simulink model "gnc"  (R2023a)
settings: Solver=ode4  StartTime=0.0  StopTime=10.0  FixedStep=dt  RelTol=1e-3
undefined symbols (not defined in the file): dt, plant, u_mat_full, u_time
libraries: aerolibutil x2
settings Model: Creator=ndelurgio  LastModifiedBy=ndelurgio

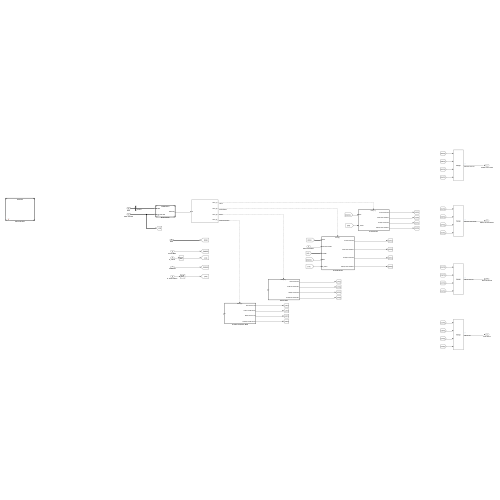
[thumbnail: Simulink's stored preview of the top-level diagram]
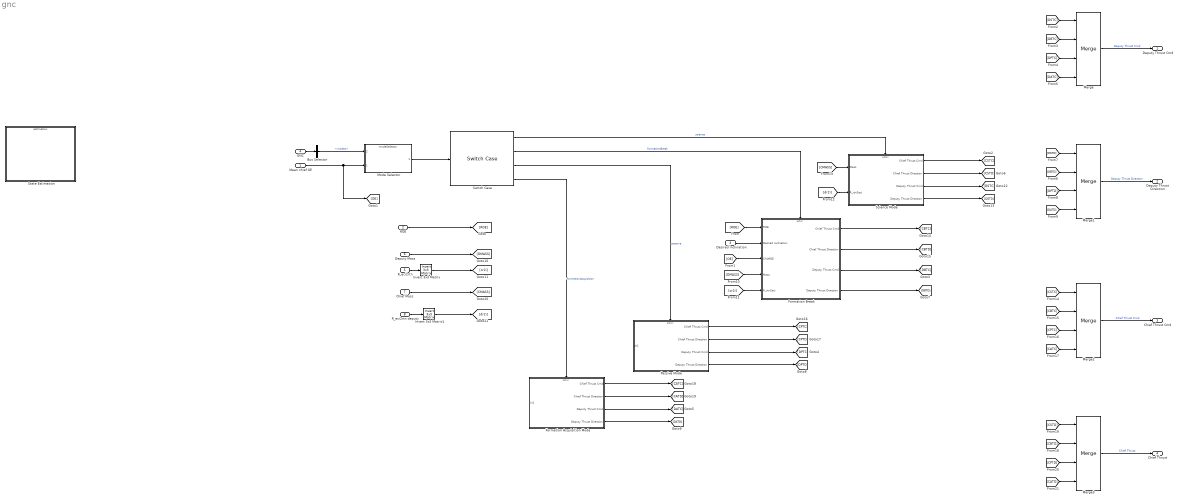
== system gnc ==
  Mean chief OE : Inport  OutDataTypeStr=Bus: meanOrbitElements
  ROE : Inport  Port=2  OutDataTypeStr=Bus: eccentricSingularROE
  Desired inclination : Inport  Port=3  PortDimensions=2
  GNC : Inport  Port=4  OutDataTypeStr=Bus: gncBus
  R_eci2rtn : Inport  Port=5  PortDimensions=[3,3]
  Deputy Mass : Inport  Port=6
  Chief Mass : Inport  Port=7
  R_eci2rtn deputy : Inport  Port=8
  Bus Selector : BusSelector  OutputSignals=modes
  Formation Acquisition Mode : Subsystem  TreatAsAtomicUnit=on
  Formation Break : Subsystem  TreatAsAtomicUnit=on
  Invert 3x3 Matrix : aerolibutil/Invert  3x3 Matrix
  Invert 3x3 Matrix1 : aerolibutil/Invert  3x3 Matrix
  Merge : Merge  Inputs=4  InitialOutput=0
  Merge1 : Merge  Inputs=4  InitialOutput=[1,1,1]
  Merge2 : Merge  Inputs=4  InitialOutput=0
  Merge3 : Merge  Inputs=4  InitialOutput=[1,1,1]
  Mode Selector : ModelReference  ModelNameDialog=modeSelector.slx  SimulationMode=Normal  ModelReferenceVersion=1.12
      settings: PortSchema="{\"entries\":[{\"content\":{\"sides\":[{\"content\":{\"connectorIds\":[\"In2\",\"In1\"]},\"type\":\"ConnectorPlacement.EquallySpacedRectSide\",\"uuid\":\"8a45dd05-9625-4267-a143-38565687985f\"},{\"content\":{\"connectorIds\":[\"Out1\"],\"side\":\"RIGHT\"},\"type\":\"ConnectorPlacement.EquallySpacedRectSide\",\"uuid\":\"c16609dd-c717-4d96-a97d-40d34aa61c5b\"},{\"content\":{\"side\":\"TOP\"},\"type\":\"ConnectorPlacement.EquallySpacedRectSide\",\"uuid\":\"265a618d-b5cc-4228-aeff-cbf882e13e2d\"}]},\"type\":\"ConnectorPlacement.EquallySpacedConnector\",\"uuid\":\"354b4fb0-049b-4d87-9ce4-a2a1b71aacc7\"}],\"packageUris\":[\"http://schema.mathworks.com/mf0/Connector/R2020b\"],\"version\":\"1.0\"}"
  Passive Mode : Subsystem  TreatAsAtomicUnit=on
  Science Mode : Subsystem  TreatAsAtomicUnit=on
  State Estimation : ModelReference  ModelNameDialog=estimation.slx  SimulationMode=Normal  ModelReferenceVersion=1.1
  Switch Case : SwitchCase  CaseConditions={1,2,3,4}  ShowDefaultCase=off
  Deputy Thrust Cmd : Outport
  Deputy Thrust Direction : Outport  Port=2
  Chief Thrust Cmd : Outport  Port=3
  Chief Thrust : Outport  Port=4
  wires:
  Mean chief OE/1 -> [OE], Mode Selector/1
  ROE/1 -> [ROE]
  Desired inclination/1 -> Formation Break/2(Desired inclination)
  Merge/1 -> Deputy Thrust Cmd/1  "Deputy Thrust Cmd"
  Merge1/1 -> Deputy Thrust Direction/1  "Deputy Thrust Direction"
  Switch Case/1 -> Science Mode/Action  "science"
  Switch Case/2 -> Formation Break/Action  "formationBreak"
  Switch Case/3 -> Passive Mode/Action  "passive"
  Switch Case/4 -> Formation Acquisition Mode/Action  "formationAcquisition"
  Mode Selector/1 -> Switch Case/1
  GNC/1 -> Bus Selector/1
  Bus Selector/1 -> Mode Selector/2  "<modes>"
  [ROE] -> Formation Break/1(ROE)
  [OE] -> Formation Break/3(ChiefOE)
  Invert 3x3 Matrix/1 -> [cr2i]
  Deputy Mass/1 -> [DMASS]
  R_eci2rtn/1 -> Invert 3x3 Matrix/1
  Science Mode/1(Chief Thrust Cmd) -> [CSTC]
  Formation Break/3(Deputy Thrust Cmd) -> [DBTC]
  Passive Mode/3(Deputy Thrust Cmd) -> [DPTC]
  Formation Acquisition Mode/3(Deputy Thrust Cmd) -> [DATC]
  [DSTC] -> Merge/1
  [DBTC] -> Merge/2
  [DPTC] -> Merge/3
  [DATC] -> Merge/4
  Science Mode/2(Chief Thrust Direction) -> [CSTD]
  Formation Break/4(Deputy Thrust Direction) -> [DBTD]
  Passive Mode/4(Deputy Thrust Direction) -> [DPTD]
  Formation Acquisition Mode/4(Deputy Thrust Direction) -> [DATD]
  [DSTD] -> Merge1/1
  [DBTD] -> Merge1/2
  [DPTD] -> Merge1/3
  [DATD] -> Merge1/4
  [DMASS] -> Formation Break/4(Mass)
  [cr2i] -> Formation Break/5(R_rtn2eci)
  [dr2i] -> Science Mode/2(R_rtn2eci)
  [CMASS] -> Science Mode/1(Mass)
  Science Mode/3(Deputy Thrust Cmd) -> [DSTC]
  Science Mode/4(Deputy Thrust Direction) -> [DSTD]
  Formation Break/2(Chief Thrust Direction) -> [CBTD]
  Formation Break/1(Chief Thrust Cmd) -> [CBTC]
  Passive Mode/1(Chief Thrust Cmd) -> [CPTC]
  Passive Mode/2(Chief Thrust Direction) -> [CPTD]
  Formation Acquisition Mode/1(Chief Thrust Cmd) -> [CATC]
  Formation Acquisition Mode/2(Chief Thrust Direction) -> [CATD]
  [CSTC] -> Merge2/1
  [CPTC] -> Merge2/3
  [CATC] -> Merge2/4
  [CBTC] -> Merge2/2
  [CSTD] -> Merge3/1
  [CBTD] -> Merge3/2
  [CATD] -> Merge3/4
  [CPTD] -> Merge3/3
  Merge3/1 -> Chief Thrust/1  "Chief Thrust"
  Merge2/1 -> Chief Thrust Cmd/1  "Chief Thrust Cmd"
  Chief Mass/1 -> [CMASS]
  R_eci2rtn deputy/1 -> Invert 3x3 Matrix1/1
  Invert 3x3 Matrix1/1 -> [dr2i]

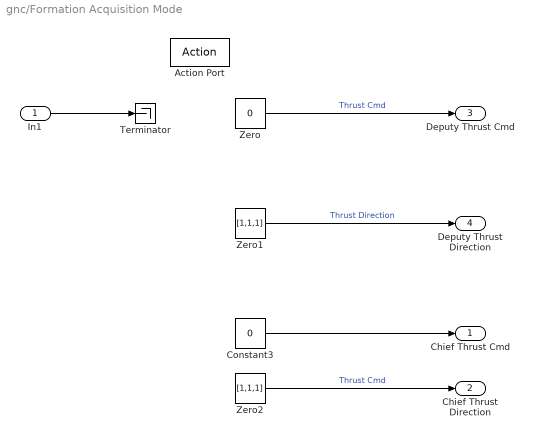
== system gnc/Formation Acquisition Mode ==
  In1 : Inport
  Action Port : ActionPort  ActionPortLabel=case [ 4 ]:
  Constant3 : Constant  Value=0
  Terminator : Terminator
  Zero : Constant  Value=0  OutDataTypeStr=Inherit: Inherit via back propagation
  Zero1 : Constant  Value=[1,1,1]  OutDataTypeStr=Inherit: Inherit via back propagation
  Zero2 : Constant  Value=[1,1,1]  OutDataTypeStr=Inherit: Inherit via back propagation
  Chief Thrust Cmd : Outport
  Chief Thrust Direction : Outport  Port=2
  Deputy Thrust Cmd : Outport  Port=3
  Deputy Thrust Direction : Outport  Port=4
  wires:
  In1/1 -> Terminator/1
  Zero/1 -> Deputy Thrust Cmd/1  "Thrust Cmd"
  Zero1/1 -> Deputy Thrust Direction/1  "Thrust Direction"
  Zero2/1 -> Chief Thrust Direction/1  "Thrust Cmd"
  Constant3/1 -> Chief Thrust Cmd/1

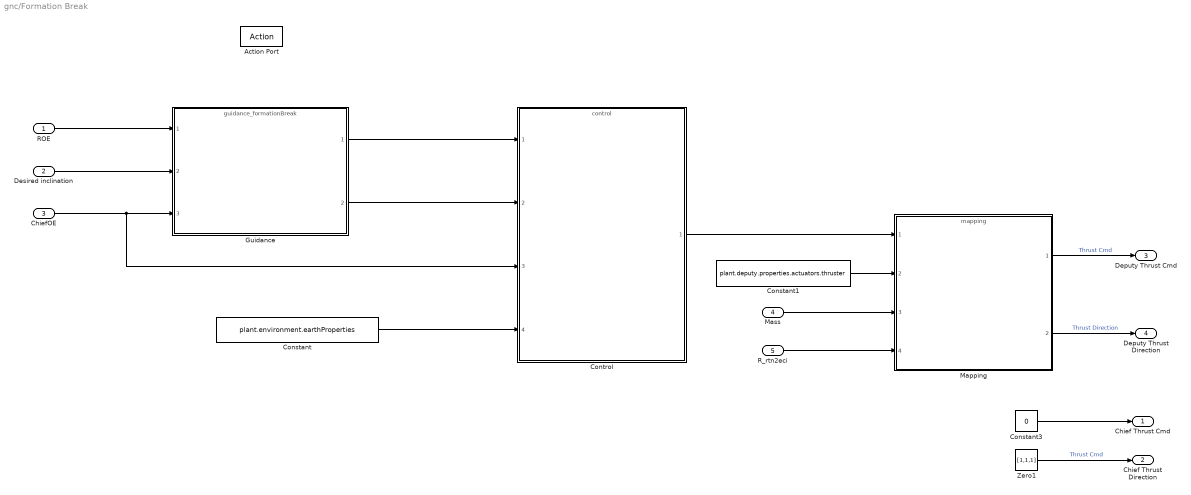
== system gnc/Formation Break ==
  ROE : Inport
  Desired inclination : Inport  Port=2
  ChiefOE : Inport  Port=3
  Mass : Inport  Port=4
  R_rtn2eci : Inport  Port=5
  Action Port : ActionPort  ActionPortLabel=case [ 2 ]:
  Constant : Constant  Value=plant.environment.earthProperties  OutDataTypeStr=Bus: earthProperties
  Constant1 : Constant  Value=plant.deputy.properties.actuators.thruster  OutDataTypeStr=Bus: thruster
  Constant3 : Constant  Value=0
  Control : ModelReference  ModelNameDialog=control.slx  SimulationMode=Normal  ModelReferenceVersion=1.13
  Guidance : ModelReference  ModelNameDialog=guidance_formationBreak  SimulationMode=Normal  ModelReferenceVersion=1.49
  Mapping : ModelReference  ModelNameDialog=mapping.slx  SimulationMode=Normal  ModelReferenceVersion=1.29
  Zero1 : Constant  Value=[1,1,1]  OutDataTypeStr=Inherit: Inherit via back propagation
  Chief Thrust Cmd : Outport
  Chief Thrust Direction : Outport  Port=2
  Deputy Thrust Cmd : Outport  Port=3
  Deputy Thrust Direction : Outport  Port=4
  wires:
  ROE/1 -> Guidance/1
  Guidance/1 -> Control/1
  Guidance/2 -> Control/2
  Desired inclination/1 -> Guidance/2
  ChiefOE/1 -> Control/3, Guidance/3
  Constant/1 -> Control/4
  Control/1 -> Mapping/1
  Constant1/1 -> Mapping/2
  Mass/1 -> Mapping/3
  R_rtn2eci/1 -> Mapping/4
  Mapping/1 -> Deputy Thrust Cmd/1  "Thrust Cmd"
  Mapping/2 -> Deputy Thrust Direction/1  "Thrust Direction"
  Constant3/1 -> Chief Thrust Cmd/1
  Zero1/1 -> Chief Thrust Direction/1  "Thrust Cmd"

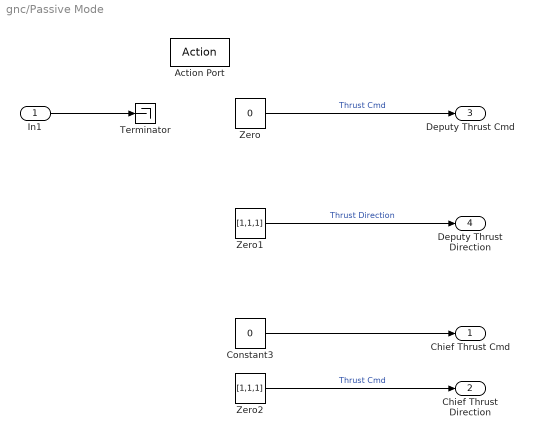
== system gnc/Passive Mode ==
  In1 : Inport
  Action Port : ActionPort  ActionPortLabel=case [ 3 ]:
  Constant3 : Constant  Value=0
  Terminator : Terminator
  Zero : Constant  Value=0  OutDataTypeStr=Inherit: Inherit via back propagation
  Zero1 : Constant  Value=[1,1,1]  OutDataTypeStr=Inherit: Inherit via back propagation
  Zero2 : Constant  Value=[1,1,1]  OutDataTypeStr=Inherit: Inherit via back propagation
  Chief Thrust Cmd : Outport
  Chief Thrust Direction : Outport  Port=2
  Deputy Thrust Cmd : Outport  Port=3
  Deputy Thrust Direction : Outport  Port=4
  wires:
  In1/1 -> Terminator/1
  Zero/1 -> Deputy Thrust Cmd/1  "Thrust Cmd"
  Zero1/1 -> Deputy Thrust Direction/1  "Thrust Direction"
  Zero2/1 -> Chief Thrust Direction/1  "Thrust Cmd"
  Constant3/1 -> Chief Thrust Cmd/1

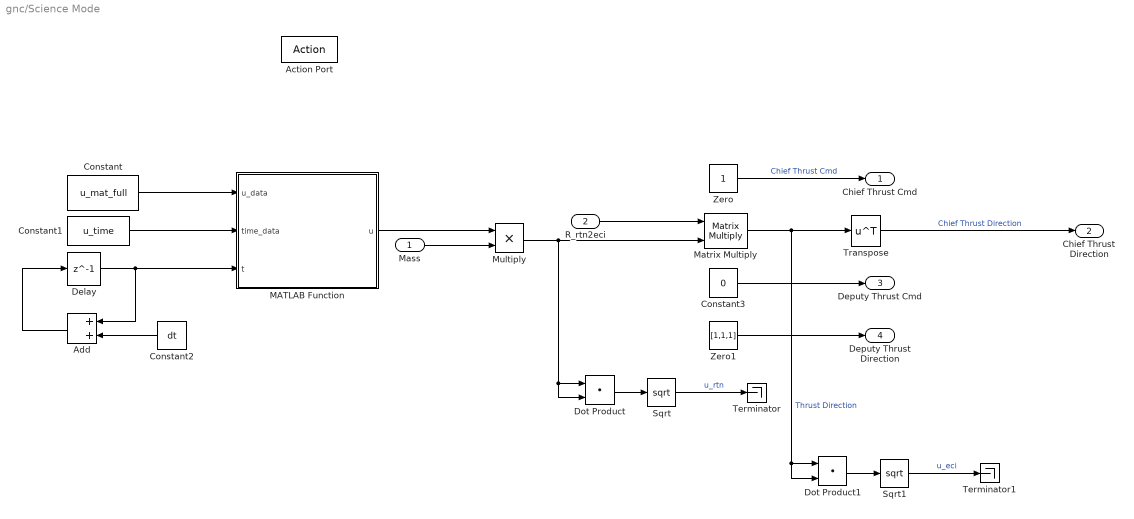
== system gnc/Science Mode ==
  Mass : Inport
  R_rtn2eci : Inport  Port=2
  Action Port : ActionPort  ActionPortLabel=case [ 1 ]:
  Add : Sum
  Constant : Constant  Value=u_mat_full
  Constant1 : Constant  Value=u_time
  Constant2 : Constant  Value=dt
  Constant3 : Constant  Value=0
  Delay : Delay  DelayLength=1
  Dot Product : DotProduct  OutDataTypeStr=Inherit: Inherit via internal rule
  Dot Product1 : DotProduct  OutDataTypeStr=Inherit: Inherit via internal rule
  MATLAB Function : MATLAB Function  TreatAsAtomicUnit=on
  Matrix Multiply : Product  Multiplication=Matrix(*)
  Multiply : Product  Inputs=**
  Sqrt : Sqrt
  Sqrt1 : Sqrt
  Terminator : Terminator
  Terminator1 : Terminator
  Transpose : Math  Operator=transpose
  Zero : Constant  OutDataTypeStr=Inherit: Inherit via back propagation
  Zero1 : Constant  Value=[1,1,1]  OutDataTypeStr=Inherit: Inherit via back propagation
  Chief Thrust Cmd : Outport
  Chief Thrust Direction : Outport  Port=2
  Deputy Thrust Cmd : Outport  Port=3
  Deputy Thrust Direction : Outport  Port=4
  wires:
  Zero/1 -> Chief Thrust Cmd/1  "Chief Thrust Cmd"
  Matrix Multiply/1 -> Dot Product1/2, Dot Product1/1, Transpose/1  "Thrust Direction"
  Constant/1 -> MATLAB Function/1(u_data)
  Constant1/1 -> MATLAB Function/2(time_data)
  Delay/1 -> Add/1, MATLAB Function/3(t)
  Constant2/1 -> Add/2
  Add/1 -> Delay/1
  MATLAB Function/1(u) -> Multiply/1
  Mass/1 -> Multiply/2
  R_rtn2eci/1 -> Matrix Multiply/1
  Multiply/1 -> Dot Product/2, Dot Product/1, Matrix Multiply/2
  Constant3/1 -> Deputy Thrust Cmd/1
  Zero1/1 -> Deputy Thrust Direction/1
  Transpose/1 -> Chief Thrust Direction/1  "Chief Thrust Direction"
  Dot Product/1 -> Sqrt/1
  Sqrt/1 -> Terminator/1  "u_rtn"
  Dot Product1/1 -> Sqrt1/1
  Sqrt1/1 -> Terminator1/1  "u_eci"

== matlab function gnc/Science Mode/MATLAB Function ==
  data: u_data input; u output; time_data input; t input
function u = getControlCmd(u_data,time_data,t)
u = getControlCmd(u_data,time_data,t);
end
